simulink model "if_else_Model"  (R2013b)
settings: Solver=ode4  StartTime=0.0  StopTime=inf  FixedStep=0.10  RelTol=1e-3
undefined symbols (not defined in the file): sigbuilder_block
libraries: simulink x1
settings Model: Creator=daltdoer  LastModifiedBy=daltdoer

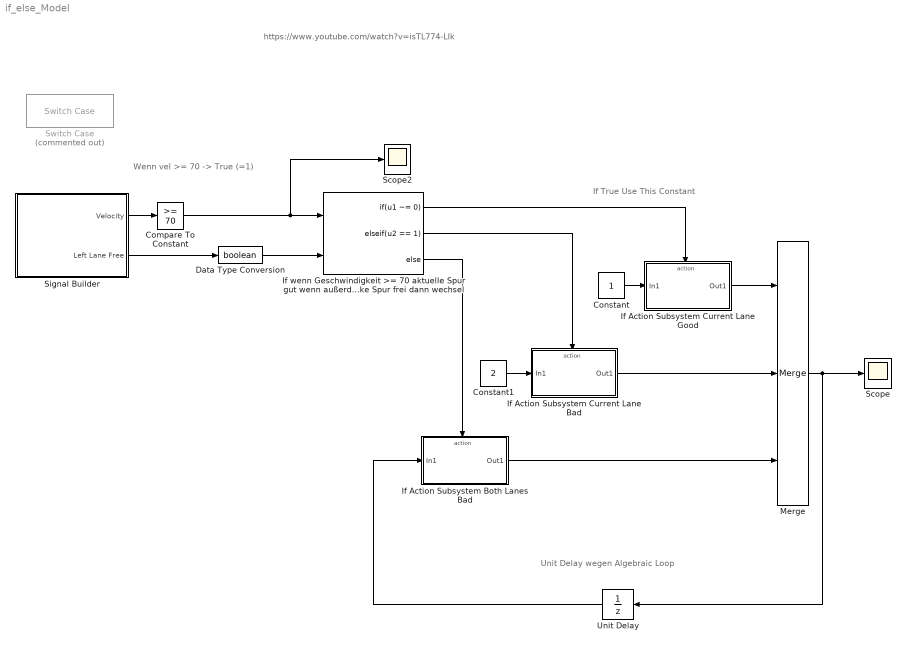
== system if_else_Model ==
  note: Unit Delay wegen Algebraic Loop
  note: If True Use This Constant
  note: Wenn vel >= 70 -> True (=1)
  note: https://www.youtube.com/watch?v=isTL774-LIk
  Compare To Constant : simulink/Logic and Bit Operations/Compare To Constant  relop=>=  const=70  OutDataTypeStr=boolean
  Constant : Constant
  Constant1 : Constant  Value=2
  Data Type Conversion : DataTypeConversion  OutDataTypeStr=boolean
  "If wenn Geschwindigkeit >= 70 aktuelle Spur gut wenn außerdem Linke Spur frei dann wechsel " : If  NumInputs=2  IfExpression=u1 ~= 0  ElseIfExpressions=u2 == 1
  If Action Subsystem Both Lanes Bad : Subsystem  TreatAsAtomicUnit=on
  If Action Subsystem Current Lane Bad : Subsystem  TreatAsAtomicUnit=on
  If Action Subsystem Current Lane Good : Subsystem  TreatAsAtomicUnit=on
  Merge : Merge  Inputs=3
  Scope : Scope
  Scope2 : Scope
      settings: SaveName=ScopeData2
  Signal Builder : Subsystem  Tag=STV Subsys  LoadFcn=sigbuilder_block('load');  StartFcn=sigbuilder_block('start');  StopFcn=sigbuilder_block('stop');  ClipboardFcn=sigbuilder_block('clipboard');  mask(Sigbuilder block){}
      mask help: Simulink:masks:SigbuilderBlock_MD
      mask init:
      | if ~strcmp(get_param(bdroot(gcbh),'SimulationStatus'),'stopped') tuvar = sigbuilder_block('maskInit'); end
      settings: CopyFcn=sigbuilder_block('copy');  DeleteFcn=sigbuilder_block('delete');  ModelCloseFcn=sigbuilder_block('modelClose');  PreSaveFcn=sigbuilder_block('preSave');  PauseFcn=sigbuilder_block('pause');  ContinueFcn=sigbuilder_block('continue');  NameChangeFcn=sigbuilder_block('namechange');  OpenFcn=sigbuilder_block('open',[417.103 80.069 543.724 428.276 ]);  CloseFcn=sigbuilder_block('close');
      mask Display: plot(0, 0, 100, 100,[2, 2, 32, 32, 2], [68, 8, 8, 68, 68],[32, 2], [38, 38], [32, 19, 2],[53, 60, 44], [32, 17, 17, 2],[16, 16, 31, 31]);txt = getActiveGroup(gcbh);text(2, 100, txt,'verticalAlignment', 'top');
  Switch Case : SwitchCase  Commented=on
  Unit Delay : UnitDelay  SampleTime=-1
  wires:
  Compare To Constant/1 -> "If wenn Geschwindigkeit >= 70 aktuelle Spur gut wenn außerdem Linke Spur frei dann wechsel "/1, Scope2/1
  ? -> Switch Case/1
  "If wenn Geschwindigkeit >= 70 aktuelle Spur gut wenn außerdem Linke Spur frei dann wechsel "/1 -> If Action Subsystem Current Lane Good/Action
  "If wenn Geschwindigkeit >= 70 aktuelle Spur gut wenn außerdem Linke Spur frei dann wechsel "/2 -> If Action Subsystem Current Lane Bad/Action
  "If wenn Geschwindigkeit >= 70 aktuelle Spur gut wenn außerdem Linke Spur frei dann wechsel "/3 -> If Action Subsystem Both Lanes Bad/Action
  Signal Builder/1(Velocity) -> Compare To Constant/1
  Signal Builder/2(Left Lane Free) -> Data Type Conversion/1
  Data Type Conversion/1 -> "If wenn Geschwindigkeit >= 70 aktuelle Spur gut wenn außerdem Linke Spur frei dann wechsel "/2
  If Action Subsystem Current Lane Good/1(Out1) -> Merge/1
  If Action Subsystem Current Lane Bad/1(Out1) -> Merge/2
  If Action Subsystem Both Lanes Bad/1(Out1) -> Merge/3
  Constant/1 -> If Action Subsystem Current Lane Good/1(In1)
  Constant1/1 -> If Action Subsystem Current Lane Bad/1(In1)
  Merge/1 -> Unit Delay/1, Scope/1
  Unit Delay/1 -> If Action Subsystem Both Lanes Bad/1(In1)

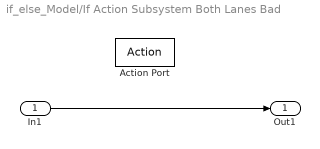
== system if_else_Model/If Action Subsystem Both Lanes Bad ==
  In1 : Inport
  Action Port : ActionPort  ActionType=else
  Out1 : Outport
  wires:
  In1/1 -> Out1/1

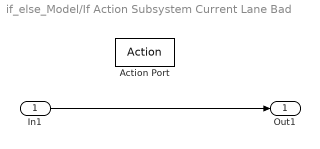
== system if_else_Model/If Action Subsystem Current Lane Bad ==
  In1 : Inport
  Action Port : ActionPort  ActionType=elseif
  Out1 : Outport
  wires:
  In1/1 -> Out1/1

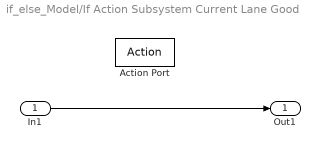
== system if_else_Model/If Action Subsystem Current Lane Good ==
  In1 : Inport
  Action Port : ActionPort  ActionType=then
  Out1 : Outport
  wires:
  In1/1 -> Out1/1

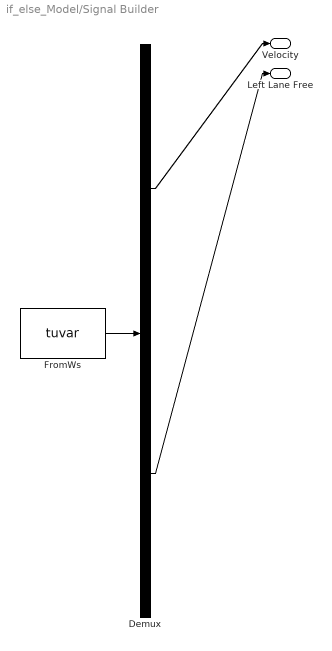
== system if_else_Model/Signal Builder ==
  Demux : Demux  Tag=STV Demux  Outputs=2
  FromWs : FromWorkspace  Tag=STV FromWs  VariableName=tuvar  SampleTime=0
      SigBuilderData=|
      | common.afterFinalStr = 'Extrapolate'
      | common.sampleTime = 0
      | dataSet.timeRange = [0 10]
      | dataSet.name = 'Group 1'
      | sbobj.Groups.Name = 'Group 1'
      | sbobj.Groups.Signals(1).Name = 'Velocity'
      | sbobj.Groups.Signals(1).XData = [0 4 4 6 6 10]
      | sbobj.Groups.Signals(1).YData = [70 70 60 60 70 70]
      | sbobj.Groups.Signals(2).Name = 'Left Lane Free'
      | sbobj.Groups.Signals(2).XData = [0 3 3 6 6 10]
      | sbobj.Groups.Signals(2).YData = [0 0 1 1 0 0]
  Velocity : Outport  Tag=STV Outport
  Left Lane Free : Outport  Tag=STV Outport  Port=2
  wires:
  FromWs/1 -> Demux/1
  Demux/1 -> Velocity/1
  Demux/2 -> Left Lane Free/1
